simulink model "RL_Heat_DDPG_test1"  (R2021b)
settings: Solver=VariableStepAuto  StartTime=0.0  StopTime=48  RelTol=1e-3
model workspace (MAT data in the model file):
  Troom = 30
undefined symbols (not defined in the file): c, cost, DiscIntNeverNeededParam, M, Mdot, Req, THeater, TinIC, Ts
libraries: simulink_extras x3, simulink x3, rllib x1
settings Model: Creator=abhijit  LastModifiedBy=mluser
settings SolverCC: AlgebraicLoopSolver=TrustRegion
settings DebuggingCC: SFMachineParentedDataDiag=warning

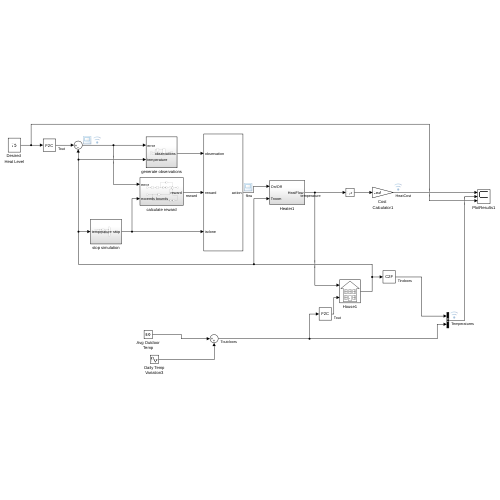
[thumbnail: Simulink's stored preview of the top-level diagram]
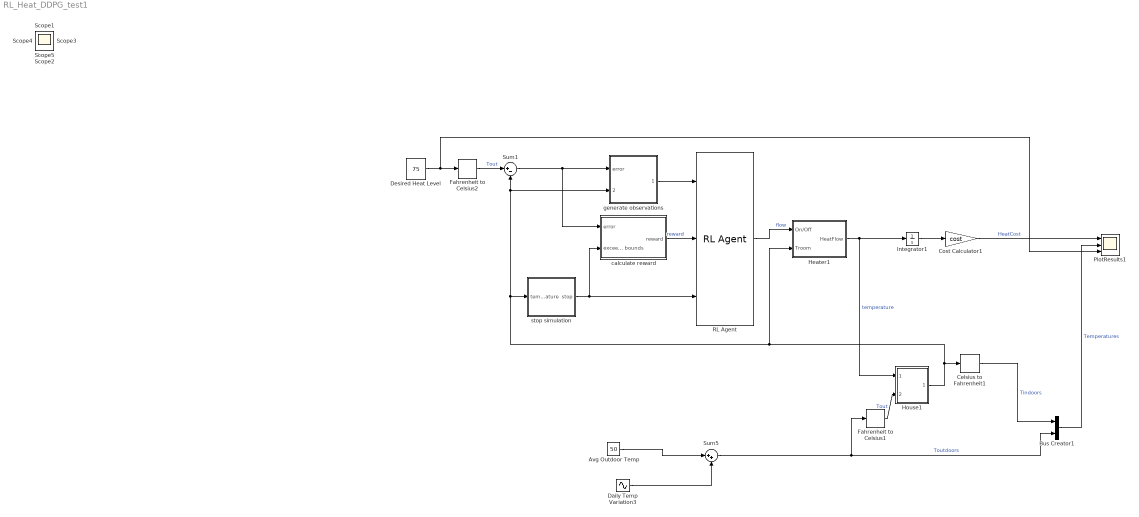
== system RL_Heat_DDPG_test1 ==
  Avg Outdoor Temp : Constant  Value=50
  Bus Creator1 : BusCreator  Inputs=2
  Celsius to Fahrenheit1 : simulink_extras/Transformations/Celsius to Fahrenheit
      settings: SourceProductBaseCode=SL
  Cost Calculator1 : Gain  Gain=cost  SaturateOnIntegerOverflow=on  OutDataTypeStr=Inherit: Same as input  ParamDataTypeStr=Inherit: Same as input
  Daily Temp Variation3 : Sin  Amplitude=15  Frequency=2*pi/24  SampleTime=0
  Desired Heat Level : Constant  Value=75
  Fahrenheit to Celsius1 : simulink_extras/Transformations/Fahrenheit to Celsius
      settings: SourceProductBaseCode=SL
  Fahrenheit to Celsius2 : simulink_extras/Transformations/Fahrenheit to Celsius
      settings: SourceProductBaseCode=SL
  Heater1 : Subsystem
  House1 : Subsystem
      mask Display: image(fullfile(matlabroot,'toolbox','simulink','simdemos','simgeneral','images','HouseHeatHousePix.svg'))
  Integrator1 : Integrator
  PlotResults1 : Scope  NumInputPorts=3
  RL Agent : rllib/RL Agent  Agent=agent  ExternalActionAsInput=off  ProvideCumRwd=off  TreatAsDirectFeedthrough=on
  Sum1 : Sum  Inputs=|+-  SaturateOnIntegerOverflow=on
  Sum5 : Sum  Inputs=|++  InputSameDT=on  SaturateOnIntegerOverflow=on  OutDataTypeStr=Inherit: Same as first input
  calculate reward : Subsystem
  generate observations : Subsystem
  stop simulation : Subsystem
  Scope{,1..5} (6 alike) : Scope
  wires:
  calculate reward/1(reward) -> RL Agent/2  "reward"
  stop simulation/1(stop) -> RL Agent/3, calculate reward/2(exceeds bounds)
  generate observations/1(observations) -> RL Agent/1
  RL Agent/1 -> Heater1/1(On/Off)  "flow"
  Sum1/1 -> calculate reward/1(error), generate observations/1(error)
  Heater1/1(HeatFlow) -> Integrator1/1, House1/1(Heater QDot In)  "temperature"
  Desired Heat Level/1 -> PlotResults1/3, Fahrenheit to Celsius2/1
  Fahrenheit to Celsius1/1 -> House1/2(Outdoor Temp Tout)  "Tout"
  Sum5/1 -> Bus Creator1/2, Fahrenheit to Celsius1/1  "Toutdoors"
  Avg Outdoor Temp/1 -> Sum5/1
  Celsius to Fahrenheit1/1 -> Bus Creator1/1  "Tindoors"
  House1/1(Room Temp Troom) -> Heater1/2(Troom), stop simulation/1(temperature), generate observations/2(temperature), Sum1/2, Celsius to Fahrenheit1/1
  Integrator1/1 -> Cost Calculator1/1
  Cost Calculator1/1 -> PlotResults1/1  "HeatCost"
  Bus Creator1/1 -> PlotResults1/2  "Temperatures"
  Fahrenheit to Celsius2/1 -> Sum1/1  "Tout"
  Daily Temp Variation3/1 -> Sum5/2

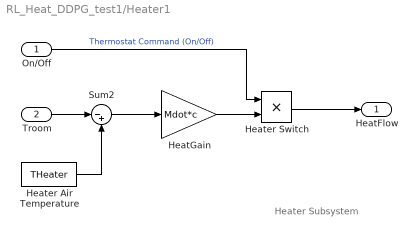
== system RL_Heat_DDPG_test1/Heater1 ==
  note: Heater Subsystem
  On/Off : Inport
  Troom : Inport  Port=2
  HeatGain : Gain  Gain=Mdot*c
  Heater Air Temperature : Constant  Value=THeater
  Heater Switch : Product  RndMeth=Zero
  Sum2 : Sum  Inputs=|-+
  HeatFlow : Outport  VectorParamsAs1DForOutWhenUnconnected=off
  wires:
  Heater Air Temperature/1 -> Sum2/2
  Troom/1 -> Sum2/1
  Sum2/1 -> HeatGain/1
  On/Off/1 -> Heater Switch/1  "Thermostat Command (On/Off)"
  HeatGain/1 -> Heater Switch/2
  Heater Switch/1 -> HeatFlow/1

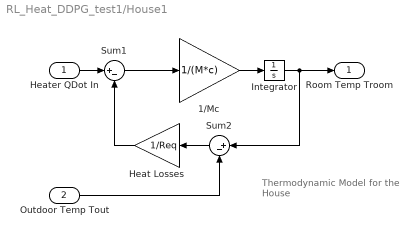
== system RL_Heat_DDPG_test1/House1 ==
  note: Thermodynamic Model
      | for the House
  Heater QDot In : Inport
  Outdoor Temp Tout : Inport  Port=2
  1/Mc : Gain  Gain=1/(M*c)  SaturateOnIntegerOverflow=on  OutDataTypeStr=Inherit: Same as input  ParamDataTypeStr=Inherit: Same as input
  Heat Losses : Gain  Gain=1/Req  SaturateOnIntegerOverflow=on  OutDataTypeStr=Inherit: Same as input  ParamDataTypeStr=Inherit: Same as input
  Integrator : Integrator  InitialCondition=TinIC
  Sum1 : Sum  Inputs=|+-  InputSameDT=on  SaturateOnIntegerOverflow=on  OutDataTypeStr=Inherit: Same as first input
  Sum2 : Sum  Inputs=|+-  InputSameDT=on  SaturateOnIntegerOverflow=on  OutDataTypeStr=Inherit: Same as first input
  Room Temp Troom : Outport  InitialOutput=0  VectorParamsAs1DForOutWhenUnconnected=off
  wires:
  Outdoor Temp Tout/1 -> Sum2/2
  Heater QDot In/1 -> Sum1/1
  Sum1/1 -> 1/Mc/1
  Sum2/1 -> Heat Losses/1
  Heat Losses/1 -> Sum1/2
  1/Mc/1 -> Integrator/1
  Integrator/1 -> Sum2/1, Room Temp Troom/1

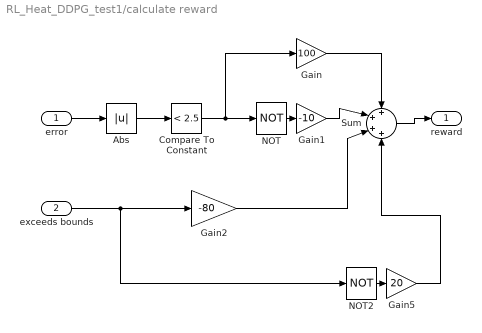
== system RL_Heat_DDPG_test1/calculate reward ==
  error : Inport
  exceeds bounds : Inport  Port=2
  Abs : Abs
  Compare To Constant : simulink/Logic and Bit Operations/Compare To Constant  relop=<  const=2.5  OutDataTypeStr=boolean
  Gain : Gain  Gain=100
  Gain1 : Gain  Gain=-10
  Gain2 : Gain  Gain=-80
  Gain5 : Gain  Gain=20
  NOT : Logic  Operator=NOT  IconShape=distinctive  AllPortsSameDT=off  OutDataTypeStr=boolean
  NOT2 : Logic  Operator=NOT  IconShape=distinctive  AllPortsSameDT=off  OutDataTypeStr=boolean
  Sum : Sum  Inputs=++++  OutDataTypeStr=double
  reward : Outport  VectorParamsAs1DForOutWhenUnconnected=off
  wires:
  Abs/1 -> Compare To Constant/1
  Gain2/1 -> Sum/3
  Gain/1 -> Sum/1
  Compare To Constant/1 -> NOT/1, Gain/1
  Gain1/1 -> Sum/2
  Sum/1 -> reward/1
  NOT/1 -> Gain1/1
  error/1 -> Abs/1
  NOT2/1 -> Gain5/1
  exceeds bounds/1 -> NOT2/1, Gain2/1
  Gain5/1 -> Sum/4

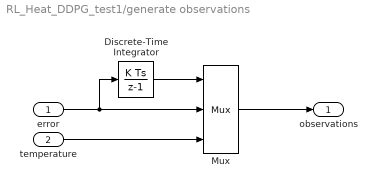
== system RL_Heat_DDPG_test1/generate observations ==
  error : Inport
  temperature : Inport  Port=2
  Discrete-Time Integrator : DiscreteIntegrator  SampleTime=Ts  ICPrevOutput=DiscIntNeverNeededParam  ICPrevScaledInput=DiscIntNeverNeededParam
  Mux : Mux  Inputs=3
  observations : Outport  VectorParamsAs1DForOutWhenUnconnected=off
  wires:
  temperature/1 -> Mux/3
  Discrete-Time Integrator/1 -> Mux/1
  error/1 -> Discrete-Time Integrator/1, Mux/2
  Mux/1 -> observations/1

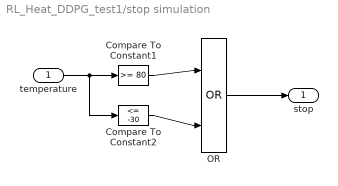
== system RL_Heat_DDPG_test1/stop simulation ==
  temperature : Inport
  Compare To Constant1 : simulink/Logic and Bit Operations/Compare To Constant  relop=>=  const=80  OutDataTypeStr=boolean
  Compare To Constant2 : simulink/Logic and Bit Operations/Compare To Constant  relop=<=  const=-30  OutDataTypeStr=boolean
  OR : Logic  Operator=OR  IconShape=distinctive  AllPortsSameDT=off  OutDataTypeStr=boolean
  stop : Outport  VectorParamsAs1DForOutWhenUnconnected=off
  wires:
  temperature/1 -> Compare To Constant2/1, Compare To Constant1/1
  Compare To Constant2/1 -> OR/2
  Compare To Constant1/1 -> OR/1
  OR/1 -> stop/1
